simulink model "simulaink_model"  (R2024a)
settings: Solver=VariableStepAuto  StartTime=0.0  StopTime=10.0  RelTol=1e-3
PreLoadFcn:
  | main
values from neighbouring files (symbols this model uses):
  attack_angle = 69    [main.m]    (also in parameter_domain_calculation.m = attack_angle_range(i_attack_angle); return_map_running.m = linspace(66, 69, 4))
  g = 9.81    [main.m]
  initial_condition = [0 ; y ; vx ; 0]    [parameter_domain_calculation.m]    (also in poincare_function_running.m = Y(:,end); poincare_function_walking.m = Y(:,end); return_map_walking.m = [x_val ; y_val ; vx_val ; vy_val]; stable_gait_calculator.m = Y(:,end))
  k = 13969.44    [main.m]    (also in parameter_domain_calculation.m = k_range(i_k); return_map_running.m = 20000; return_map_walking.m)
  leg_length = 1    [main.m]
  mass = 80    [main.m]
  phase = 1    [main.m]    (also in parameter_domain_calculation.m; poincare_function_running.m; poincare_function_walking.m; return_map_running.m = 0)
  y_land = leg_length*sind(attack_angle)    [main.m]    (also in poincare_function_running.m = Y(2,end); return_map_running.m = leg_length*sind(current_attack_angle))
settings Model: Creator=athar  LastModifiedBy=athar

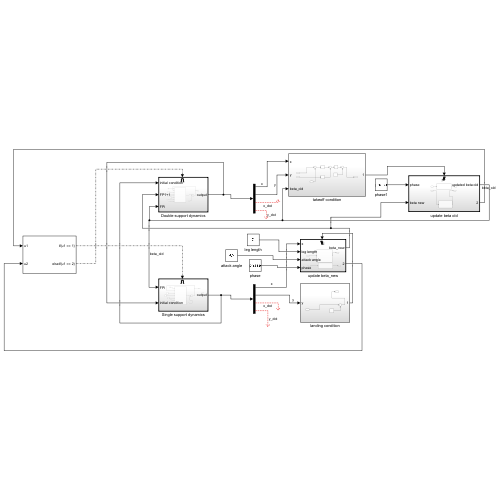
[thumbnail: Simulink's stored preview of the top-level diagram]
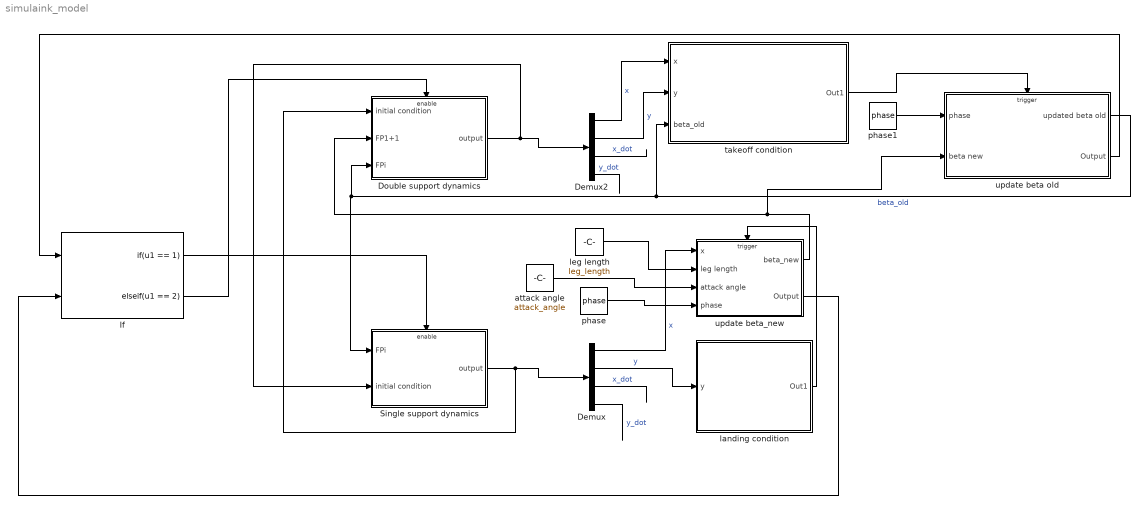
== system simulaink_model ==
  Demux : Demux
  Demux2 : Demux
  Double support dynamics : Subsystem  TreatAsAtomicUnit=on
  If : If  NumInputs=2  IfExpression=u1 == 1  ElseIfExpressions=u1 == 2  ShowElse=off
  Single support dynamics : Subsystem  TreatAsAtomicUnit=on
  attack angle : Constant  Value=attack_angle
  landing condition : Subsystem
  leg length : Constant  Value=leg_length
  phase : Constant  Value=phase
  phase1 : Constant  Value=phase
  takeoff condition : Subsystem
  update beta old : Subsystem  TreatAsAtomicUnit=on
  update beta_new : Subsystem  TreatAsAtomicUnit=on
  wires:
  Demux/1 -> update beta_new/1(x)  "x"
  Demux/3 -> ?  "x_dot"
  Demux/4 -> ?  "y_dot"
  update beta old/1(updated beta old) -> takeoff condition/3(beta_old), Single support dynamics/1(FPi), Double support dynamics/3(FPi)  "beta_old"
  Single support dynamics/1(output) -> Double support dynamics/1(initial condition), Demux/1
  leg length/1 -> update beta_new/2(leg length)
  attack angle/1 -> update beta_new/3(attack angle)
  update beta_new/1(beta_new) -> update beta old/2(beta new), Double support dynamics/2(FP1+1)
  Demux2/4 -> ?  "y_dot"
  Demux2/3 -> ?  "x_dot"
  Double support dynamics/1(output) -> Single support dynamics/2(initial condition), Demux2/1
  Demux2/1 -> takeoff condition/1(x)  "x"
  Demux2/2 -> takeoff condition/2(y)  "y"
  takeoff condition/1(Out1) -> update beta old/Trigger
  Demux/2 -> landing condition/1(y)  "y"
  landing condition/1(Out1) -> update beta_new/Trigger
  phase/1 -> update beta_new/4(phase)
  phase1/1 -> update beta old/1(phase)
  If/2 -> Double support dynamics/Enable
  update beta old/2(Output) -> If/1
  update beta_new/2(Output) -> If/2
  If/1 -> Single support dynamics/Enable

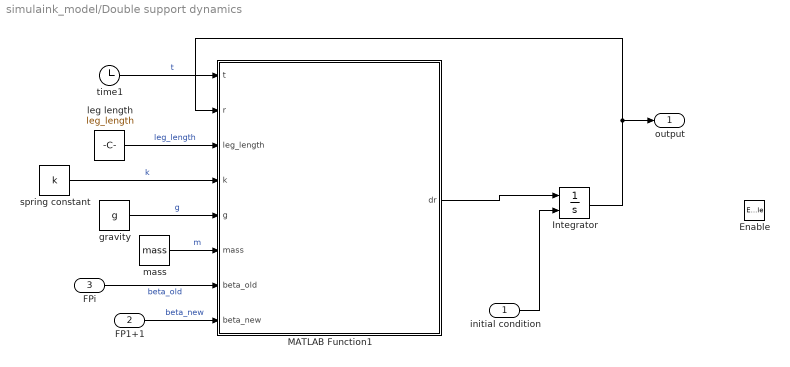
== system simulaink_model/Double support dynamics ==
  initial condition : Inport
  FP1+1 : Inport  Port=2
  FPi : Inport  Port=3
  Enable : EnablePort
  Integrator : Integrator  InitialConditionSource=external  InitialCondition=initial_condition
  MATLAB Function1 : MATLAB Function  TreatAsAtomicUnit=on
  gravity : Constant  Value=g
  leg length : Constant  Value=leg_length
  mass : Constant  Value=mass
  spring constant : Constant  Value=k
  time1 : Clock
  output : Outport
  wires:
  mass/1 -> MATLAB Function1/6(mass)  "m"
  leg length/1 -> MATLAB Function1/3(leg_length)  "leg_length"
  time1/1 -> MATLAB Function1/1(t)  "t"
  Integrator/1 -> output/1, MATLAB Function1/2(r)
  spring constant/1 -> MATLAB Function1/4(k)  "k"
  gravity/1 -> MATLAB Function1/5(g)  "g"
  MATLAB Function1/1(dr) -> Integrator/1
  FPi/1 -> MATLAB Function1/7(beta_old)  "beta_old"
  FP1+1/1 -> MATLAB Function1/8(beta_new)  "beta_new"
  initial condition/1 -> Integrator/2

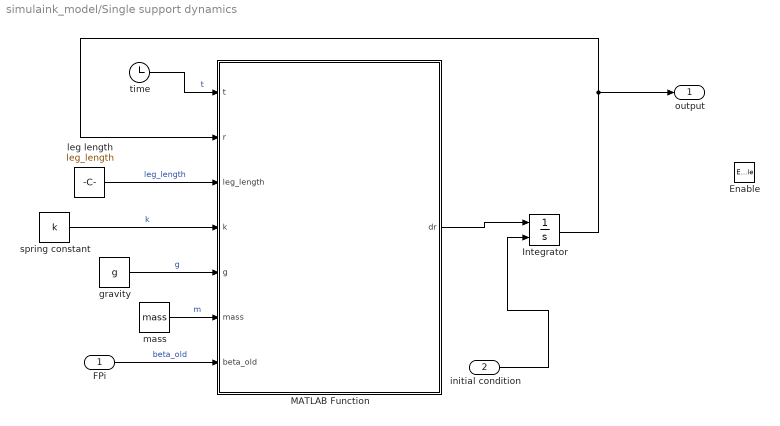
== system simulaink_model/Single support dynamics ==
  FPi : Inport
  initial condition : Inport  Port=2
  Enable : EnablePort
  Integrator : Integrator  InitialConditionSource=external
  MATLAB Function : MATLAB Function  TreatAsAtomicUnit=on
  gravity : Constant  Value=g
  leg length : Constant  Value=leg_length
  mass : Constant  Value=mass
  spring constant : Constant  Value=k
  time : Clock
  output : Outport
  wires:
  leg length/1 -> MATLAB Function/3(leg_length)  "leg_length"
  time/1 -> MATLAB Function/1(t)  "t"
  gravity/1 -> MATLAB Function/5(g)  "g"
  MATLAB Function/1(dr) -> Integrator/1
  mass/1 -> MATLAB Function/6(mass)  "m"
  FPi/1 -> MATLAB Function/7(beta_old)  "beta_old"
  spring constant/1 -> MATLAB Function/4(k)  "k"
  Integrator/1 -> MATLAB Function/2(r), output/1
  initial condition/1 -> Integrator/2

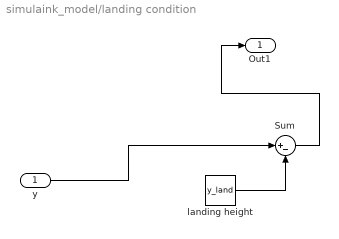
== system simulaink_model/landing condition ==
  y : Inport
  Sum : Sum  Inputs=|+-
  landing height : Constant  Value=y_land
  Out1 : Outport
  wires:
  landing height/1 -> Sum/2
  Sum/1 -> Out1/1
  y/1 -> Sum/1

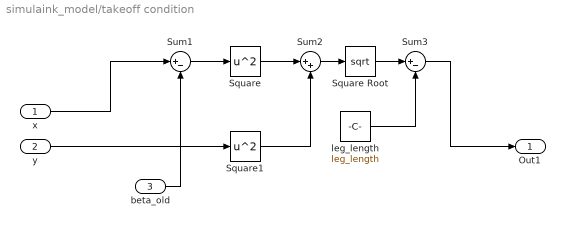
== system simulaink_model/takeoff condition ==
  x : Inport
  y : Inport  Port=2
  beta_old : Inport  Port=3
  Square : Math  Operator=square
  Square Root : Sqrt
  Square1 : Math  Operator=square
  Sum1 : Sum  Inputs=|+-
  Sum2 : Sum  Inputs=|++
  Sum3 : Sum  Inputs=|+-
  leg_length : Constant  Value=leg_length
  Out1 : Outport
  wires:
  beta_old/1 -> Sum1/2
  Sum2/1 -> Square Root/1
  Square/1 -> Sum2/1
  Sum3/1 -> Out1/1
  Sum1/1 -> Square/1
  y/1 -> Square1/1
  Square1/1 -> Sum2/2
  leg_length/1 -> Sum3/2
  x/1 -> Sum1/1
  Square Root/1 -> Sum3/1

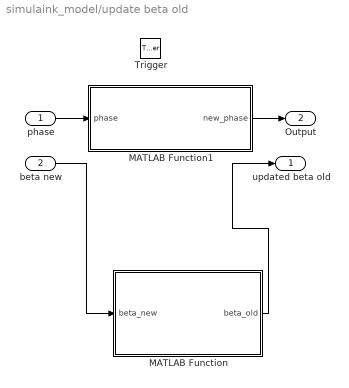
== system simulaink_model/update beta old ==
  phase : Inport
  beta new : Inport  Port=2
  Trigger : TriggerPort  VariantControl=(inherit)
  MATLAB Function : MATLAB Function  TreatAsAtomicUnit=on
  MATLAB Function1 : MATLAB Function  TreatAsAtomicUnit=on
  updated beta old : Outport  InitialOutput=0
  Output : Outport  Port=2
  wires:
  beta new/1 -> MATLAB Function/1(beta_new)
  MATLAB Function/1(beta_old) -> updated beta old/1
  phase/1 -> MATLAB Function1/1(phase)
  MATLAB Function1/1(new_phase) -> Output/1

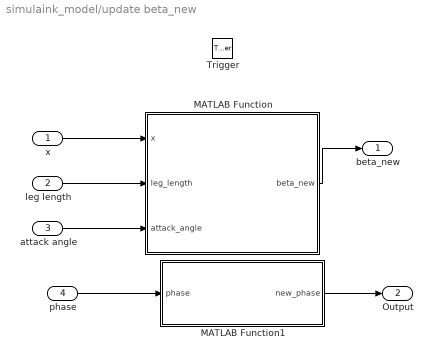
== system simulaink_model/update beta_new ==
  x : Inport
  leg length : Inport  Port=2
  attack angle : Inport  Port=3
  phase : Inport  Port=4
  Trigger : TriggerPort  TriggerType=falling  VariantControl=(inherit)
  MATLAB Function : MATLAB Function  TreatAsAtomicUnit=on
  MATLAB Function1 : MATLAB Function  TreatAsAtomicUnit=on
  beta_new : Outport
  Output : Outport  Port=2
  wires:
  MATLAB Function/1(beta_new) -> beta_new/1
  x/1 -> MATLAB Function/1(x)
  leg length/1 -> MATLAB Function/2(leg_length)
  attack angle/1 -> MATLAB Function/3(attack_angle)
  phase/1 -> MATLAB Function1/1(phase)
  MATLAB Function1/1(new_phase) -> Output/1

== matlab function simulaink_model/Double support dynamics/MATLAB Function1 ==
  data: t input; dr output; r input; leg_length input; k input; g input; mass input; beta_old input; beta_new input
function dr = double_support_dynamics(t,r,leg_length,k,g,mass,beta_old,beta_new)

x = r(1);
y = r(2);

x_dot = r(3);
y_dot = r(4);

velocity = [x_dot;y_dot];

d = beta_new - beta_old;

p = (k/mass)*(-1 + leg_length/sqrt((x - beta_old)^2 + y^2));

q = (k/mass)*(-1 + leg_length/sqrt((x - d - beta_old)^2 + y^2));
        
x_ddot_s = p*(x - beta_old) + q*(x - d - beta_old);
y_ddot_s = -g + p*y + q*y;

acceleration = [x_ddot_s;y_ddot_s];

dr = [velocity;acceleration];

end

== matlab function simulaink_model/update beta_new/MATLAB Function ==
  data: x input; beta_new output; leg_length input; attack_angle input
function beta_new = calc_beta_new(x,leg_length,attack_angle)

    beta_new = x + leg_length*cosd(attack_angle);

    phase = 2;  % Switch to double support phase

end

== matlab function simulaink_model/Single support dynamics/MATLAB Function ==
  data: t input; r input; dr output; leg_length input; k input; g input; mass input; beta_old input
function dr = single_support_dynamics(t,r,leg_length,k,g,mass,beta_old)

x = r(1);
y = r(2);

x_dot = r(3);
y_dot = r(4);

velocity = [x_dot;y_dot];

p = (k/mass)*(-1 + leg_length/sqrt((x - beta_old)^2 + y^2));
        
x_ddot_s = p*(x - beta_old);
y_ddot_s = -g + p*y;

acceleration = [x_ddot_s;y_ddot_s];

dr = [velocity;acceleration];

end

== matlab function simulaink_model/update beta old/MATLAB Function ==
  data: beta_new input; beta_old output
function beta_old   = fcn(beta_new)

beta_old = beta_new;

phase_new = phase_old - 1;

end

== matlab function simulaink_model/update beta_new/MATLAB Function1 ==
  data: phase input; new_phase output
function new_phase = updatePhase(phase)

    gain = 2;
    new_phase = phase * gain;
    assignin('base', 'phase', new_phase); % Update 'phase' in the base workspace
end

== matlab function simulaink_model/update beta old/MATLAB Function1 ==
  data: phase input; new_phase output
function new_phase = updatePhase(phase)

    gain = 0.5;
    new_phase = phase * gain;
    assignin('base', 'phase', new_phase); % Update 'phase' in the base workspace
end
